simulink model "untitled"  (R2018a)
settings: Solver=FixedStepAuto  StartTime=0.0  StopTime=100  RelTol=1e-3  EnableMultiTasking=on
libraries: dspsrcs4 x2, stm32f769ilib x1
settings Model: SimulationMode=external  Creator=hpong  LastModifiedBy=hpong
settings OptimizationCC: EnhancedBackFolding=on  PassReuseOutputArgsAs=Individual arguments  MaxStackSize=64  OptimizeBlockOrder=speed  DifferentSizesBufferReuse=on  OptimizationCustomize=off
settings DebuggingCC: ParameterTunabilityLossMsg=error
settings HardwareCC: ProdBitPerPointer=32  ProdBitPerSizeT=32  ProdBitPerPtrDiffT=32  ProdLargestAtomicInteger=Long  ProdLargestAtomicFloat=Double  ProdWordSize=32  ProdHWDeviceType=ARM Compatible->ARM Cortex
settings SFSimCC: MATLABDynamicMemAlloc=off
settings RTWCC: SystemTargetFile=ert.tlc  HardwareBoard=STM32F769I-Discovery  TLCOptions=-aInlineSetEventsForThisBaseRateFcn=TLC_FALSE -aSuppressMultiTaskScheduler=TLC_FALSE -aRateBasedStepFcn=1  TemplateMakefile=ert_default_tmf  GenerateReport=on  Toolchain=GNU Tools for ARM Embedded Processors  IncludeHyperlinkInReport=on  LaunchReport=on  GenerateTraceInfo=on  GenerateTraceReport=on  GenerateTraceReportSl=on  GenerateTraceReportSf=on  GenerateTraceReportEml=on
settings CodeAppCC: ForceParamTrailComments=on  IgnoreCustomStorageClasses=off  OperatorAnnotations=on  SimulinkDataObjDesc=on  SFDataObjDesc=on  InsertBlockDesc=on
settings ERTTargetCC: CodeReplacementLibrary=ARM Cortex-M (CMSIS)

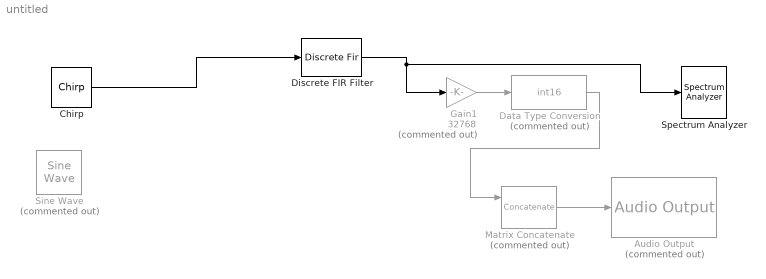
== system untitled ==
  Audio Output : stm32f769ilib/Audio Output  Commented=on  OutputDevice=Headphone  SamplingFreq=48000  Volume=62
      settings: SourceProductName=Embedded Coder Support Package for STMicroelectronics Discovery Boards  SourceProductBaseCode=STMICRODIS
  Chirp : dspsrcs4/Chirp  sweep=Linear  mode=Unidirectional  f0=0  f1=24000  t1=1  Tsweep=1  phase=0  Ts=1/48000  spf=1  datatype=Double  OutputFrames=off
      settings: SourceProductName=DSP System Toolbox
  Data Type Conversion : DataTypeConversion  Commented=on  OutDataTypeStr=int16
  Discrete FIR Filter : DiscreteFir  FilterStructure=Direct form symmetric  Coefficients="[-0.000000000000000001  -0.000151736247469566  -0.000250124091483331  -0.000256243912145059  -0.000163110002697806  0.000000000000000002  0.000175585245977243  0.000296704159812754  0.000311038307905544  0.000202190675040176  -0.000000000000000001  -0.000225521513210103  -0.000386633689770521  -0.000410335346692183  -0.000269497379461931  -0.000000000000000001  0.000305158053792129  0.000525839273443431  0.000560148646218974  0.000368804862463352  -0.000000000000000001  -0.000418400596874018  -0.000720759916485401  -0.000767046688943546  -0.000504259487376214  0.000000000000000005  0.000569592059829808  0.000978602429393342  0.001038431655053153  0.000680567269746741  -0.000000000000000002  -0.000763736153103138  -0.001307735827622802  -0.001382969325617429  -0.000903283497428826  -0.000000000000000003  0.001006841675566082  0.001718298987830316  0.001811252175713091  0.001179260153490955  -0.000000000000000003  -0.001306456794770982  -0.002223146331960839  -0.002336834731062580  -0.001517347103665295  0.000000000000000013  0.001672513534265047  0.002839349838989998  0.002977886613374269  0.001929517893652728  -0.000000000000000004  -0.002118700467477526  -0.003590657028739948  -0.003759917017202334  -0.002432739231138608  0.000000000000000005  0.002664779492668884  0.004511675851265414  0.004720456048125016  0.003052214258321956  -0.000000000000000005  -0.003340688874865114  -0.005655368588967580  -0.005917535271396478  -0.003827329673512742  0.000000000000000006  0.004194265430952493  0.007107354438139760  0.007446112656144655  0.004823352932857132  -0.000000000000000006  -0.005306946873471338  -0.009015520075398312  -0.009472728293676506  -0.006156612425203159  0.000000000000000007  0.006829083935087305  0.011658219401144636  0.012317380354050838  0.008055623253792396  -0.000000000000000007  -0.009070975874902966  -0.015626080682501330  -0.016679822445833825  -0.011036778685259315  0.000000000000000007  0.012788925774925847  0.022423266624058445  0.024431489714597823  0.016559120073362625  -0.000000000000000008  -0.020424709339336870  -0.037323264618458724  -0.042801164916056234  -0.030952787060137873  0.000000000000000008  0.046640793805924681  0.100781993932302985  0.151344740154806645  0.187199846983200940  0.200154454908176516  0.187199846983200940  0.151344740154806645  0.100781993932302985  0.046640793805924681  0.000000000000000008  -0.030952787060137873  -0.042801164916056234  -0.037323264618458724  -0.020424709339336870  -0.000000000000000008  0.016559120073362625  0.024431489714597823  0.022423266624058445  0.012788925774925847  0.000000000000000007  -0.011036778685259315  -0.016679822445833825  -0.015626080682501330  -0.009070975874902966  -0.000000000000000007  0.008055623253792396  0.012317380354050838  0.011658219401144636  0.006829083935087305  0.000000000000000007  -0.006156612425203159  -0.009472728293676506  -0.009015520075398312  -0.005306946873471338  -0.000000000000000006  0.004823352932857132  0.007446112656144655  0.007107354438139760  0.004194265430952493  0.000000000000000006  -0.003827329673512742  -0.005917535271396478  -0.005655368588967580  -0.003340688874865114  -0.000000000000000005  0.003052214258321956  0.004720456048125016  0.004511675851265414  0.002664779492668884  0.000000000000000005  -0.002432739231138608  -0.003759917017202334  -0.003590657028739948  -0.002118700467477526  -0.000000000000000004  0.001929517893652728  0.002977886613374269  0.002839349838989998  0.001672513534265047  0.000000000000000013  -0.001517347103665295  -0.002336834731062580  -0.002223146331960839  -0.001306456794770982  -0.000000000000000003  0.001179260153490955  0.001811252175713091  0.001718298987830316  0.001006841675566082  -0.000000000000000003  -0.000903283497428826  -0.001382969325617429  -0.001307735827622802  -0.000763736153103138  -0.000000000000000002  0.000680567269746741  0.001038431655053153  0.000978602429393342  0.000569592059829808  0.000000000000000005  -0.000504259487376214 ...(+542 chars)  ]"  InputProcessing=Columns as channels (frame based)  OutDataTypeStr=Inherit: Same as input
  Gain1 : Gain  Commented=on  Gain=32768
  Matrix Concatenate : Concatenate  Commented=on  Mode=Multidimensional array  ConcatenateDimension=2
  Sine Wave : dspsrcs4/Sine Wave  Commented=on  Amplitude=1  Frequency=600  Phase=0  SampleMode=Discrete  OutComplex=Real  CompMethod=Trigonometric fcn  TableSize=Speed  SampleTime=1/48000  SamplesPerFrame=12  ResetState=Restart at time zero  OutputFrames=off  dataType=Inherit via back propagation  wordLen=16  udDataType=sfix(16)  fracBitsMode=Best precision  numFracBits=15  OutDataTypeStr=Inherit: Inherit via back propagation  LastOutDataTypeStr=Inherit: Inherit via back propagation
  Spectrum Analyzer : SpectrumAnalyzer
  wires:
  Discrete FIR Filter/1 -> Spectrum Analyzer/1, Gain1/1
  Gain1/1 -> Data Type Conversion/1
  Matrix Concatenate/1 -> Audio Output/1
  Data Type Conversion/1 -> Matrix Concatenate/1
  Chirp/1 -> Discrete FIR Filter/1
